simulink model "board_fullstate_lab5"  (R2015a)
settings: Solver=ode3  StartTime=0.0  StopTime=inf  FixedStep=0.001  RelTol=1e-3
undefined symbols (not defined in the file or in its folder): A, frequency, Kx, Kxi, Ky, Kyi, ref, ref_2, ref_3, T1gain, T1offset, T2gain, T2offset, Xtare_raw, Xtare_real, Ytare_raw, Ytare_real
libraries: PoliArd x12, simulink_extras x1, dspsigops x1
settings Model: ExtModeTrigDuration=2  Creator=User  LastModifiedBy=eduar
settings OptimizationCC: OptimizeModelRefInitCode=on  LifeSpan=1
settings DebuggingCC: UnderspecifiedInitializationDetection=Classic  MergeDetectMultiDrivingBlocksExec=none
settings HardwareCC: ProdLargestAtomicInteger=Long  ProdLargestAtomicFloat=Double  ProdEndianess=LittleEndian  ProdHWDeviceType=ARM Compatible->ARM Cortex
settings RTWCC: SystemTargetFile=realtime.tlc  GenerateMakefile=off  TemplateMakefile=realtime.tmf  Description=Run on Target Hardware  RTWVerbose=off
settings ERTTargetCC: CombineOutputUpdateFcns=off  ExtModeTransport=3  ExtModeMexFile=ext_serial_win32_comm_rtt  ExtModeMexArgs=0 1 9600  InlinedParameterPlacement=Hierarchical  ERTSrcFileBannerTemplate=realtime_code_template.cgt  ERTHdrFileBannerTemplate=realtime_code_template.cgt  ERTDataSrcFileTemplate=realtime_code_template.cgt  ERTDataHdrFileTemplate=realtime_code_template.cgt  ERTCustomFileTemplate=realtime_file_process.tlc

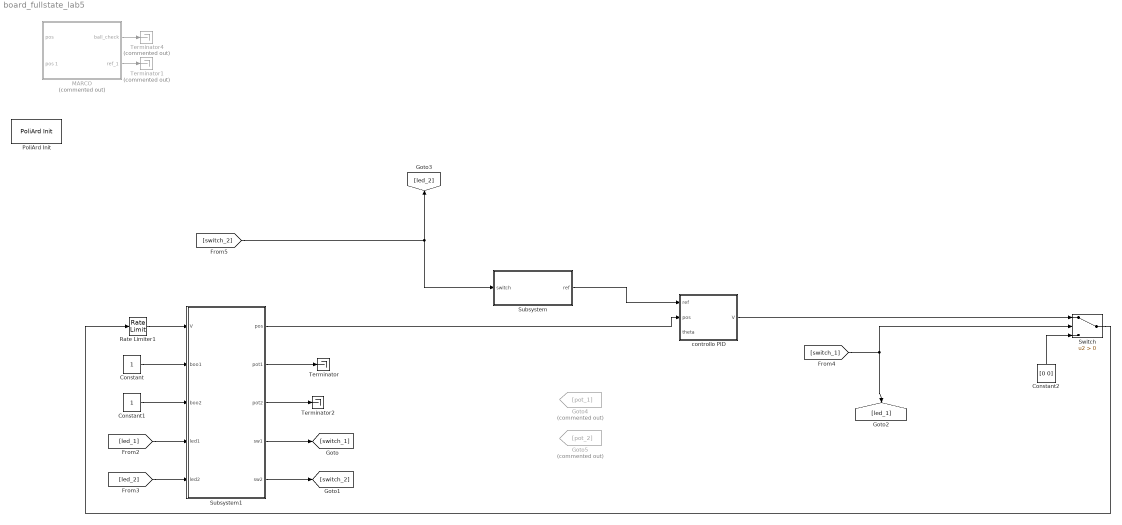
== system board_fullstate_lab5 ==
  Constant : Constant  OutDataTypeStr=boolean  SampleTime=0.01
  Constant1 : Constant  OutDataTypeStr=boolean  SampleTime=0.01
  Constant2 : Constant  Value=[0 0]  SampleTime=0.01
  Goto4 : Goto  Commented=on  GotoTag=pot_1
  Goto5 : Goto  Commented=on  GotoTag=pot_2
  MARCO : Subsystem  Commented=on
  PoliArd Init : PoliArd/PoliArd Init
  Rate Limiter1 : RateLimiter  RisingSlewLimit=20  FallingSlewLimit=-20  SampleTimeMode=inherited
  Subsystem : Subsystem
  Subsystem1 : Subsystem
  Switch : Switch  Criteria=u2 > Threshold
  Terminator : Terminator
  Terminator1 : Terminator  Commented=on
  Terminator2 : Terminator
  Terminator4 : Terminator  Commented=on
  controllo PID : Subsystem  SystemSampleTime=0.01
  wires:
  Subsystem1/1("pos ") -> controllo PID/2("pos ")
  Subsystem1/4(sw1) -> [switch_1]
  Subsystem1/5(sw2) -> [switch_2]
  [led_1] -> Subsystem1/4("led1 ")
  Constant/1 -> Subsystem1/2(boo1)
  Constant1/1 -> Subsystem1/3(boo2)
  [led_2] -> Subsystem1/5(led2)
  MARCO/2(ref_1) -> Terminator1/1
  [switch_1] -> Switch/2, [led_1]
  MARCO/1(ball_check) -> Terminator4/1
  Constant2/1 -> Switch/3
  controllo PID/1(V) -> Switch/1
  Switch/1 -> Rate Limiter1/1
  Rate Limiter1/1 -> Subsystem1/1(V)
  Subsystem1/3(pot2) -> Terminator2/1
  Subsystem1/2(pot1) -> Terminator/1
  [switch_2] -> [led_2], Subsystem/1("switch ")
  Subsystem/1("ref ") -> controllo PID/1("ref ")

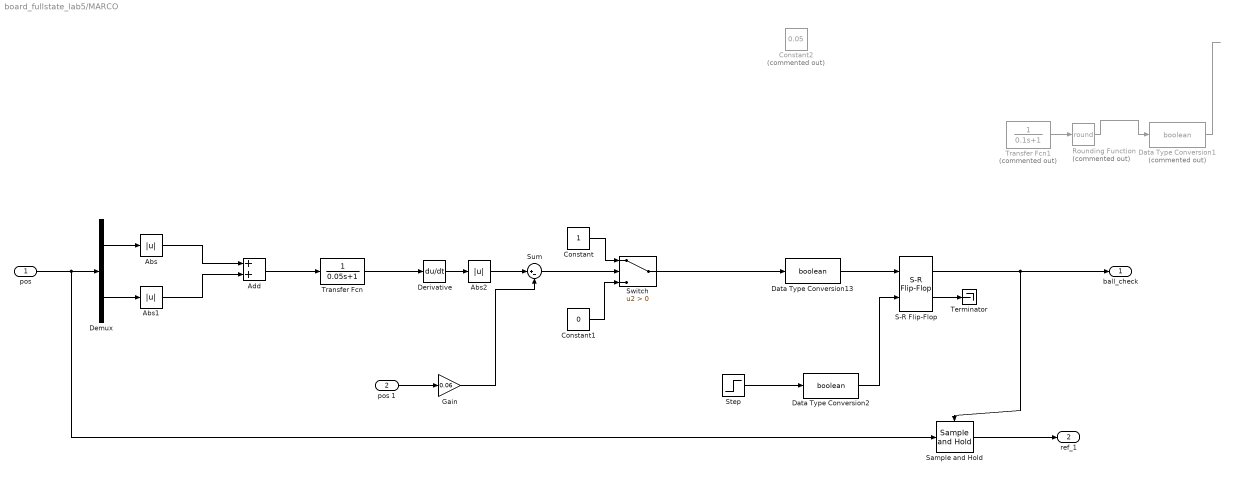
== system board_fullstate_lab5/MARCO ==
  "pos " : Inport
  pos 1 : Inport  Port=2
  Abs : Abs
  Abs1 : Abs
  Abs2 : Abs
  Add : Sum
  Constant : Constant
  Constant1 : Constant  Value=0
  Constant2 : Constant  Commented=on  Value=0.05
  Data Type Conversion1 : DataTypeConversion  Commented=on  OutDataTypeStr=boolean
  Data Type Conversion13 : DataTypeConversion  OutDataTypeStr=boolean
  Data Type Conversion2 : DataTypeConversion  OutDataTypeStr=boolean
  Demux : Demux  Outputs=2
  Derivative : Derivative
  Gain : Gain  Gain=0.06
  Rounding Function : Rounding  Commented=on  Operator=round
  S-R Flip-Flop : simulink_extras/Flip Flops/S-R Flip-Flop  initial_condition=0
  Sample and Hold : dspsigops/Sample and Hold  trig=Rising edge  initCond=0  latchinput=off
  Step : Step  Before=1  After=0
  Sum : Sum  Inputs=|+-
  Switch : Switch  Criteria=u2 > Threshold
  Terminator : Terminator
  Transfer Fcn : TransferFcn  Denominator=[0.05 1]
  Transfer Fcn1 : TransferFcn  Commented=on  Denominator=[0.1 1]
  ball_check : Outport
  ref_1 : Outport  Port=2
  wires:
  "pos "/1 -> Sample and Hold/1, Demux/1
  Demux/1 -> Abs/1
  Demux/2 -> Abs1/1
  Abs1/1 -> Add/2
  Abs/1 -> Add/1
  Derivative/1 -> Abs2/1
  Abs2/1 -> Sum/1
  Sum/1 -> Switch/2
  Constant/1 -> Switch/1
  Constant1/1 -> Switch/3
  Sample and Hold/1 -> ref_1/1
  Add/1 -> Transfer Fcn/1
  Transfer Fcn/1 -> Derivative/1
  Gain/1 -> Sum/2
  S-R Flip-Flop/1 -> ball_check/1, Sample and Hold/Trigger
  S-R Flip-Flop/2 -> Terminator/1
  Data Type Conversion13/1 -> S-R Flip-Flop/1
  Switch/1 -> Data Type Conversion13/1
  Transfer Fcn1/1 -> Rounding Function/1
  Rounding Function/1 -> Data Type Conversion1/1
  ? -> Transfer Fcn1/1
  Data Type Conversion1/1 -> ?
  Data Type Conversion2/1 -> S-R Flip-Flop/2
  Step/1 -> Data Type Conversion2/1
  pos 1/1 -> Gain/1

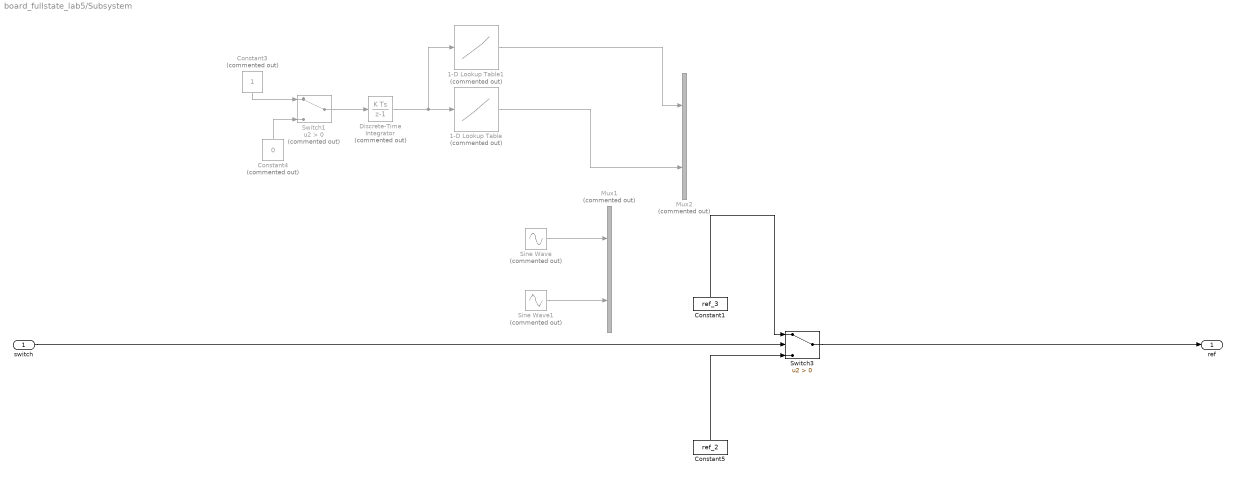
== system board_fullstate_lab5/Subsystem ==
  "switch " : Inport
  1-D Lookup Table : Lookup_n-D  Commented=on  NumberOfTableDimensions=1  BreakpointsForDimension1=ref.y.t  Table=ref.y.v  InternalRulePriority=Speed  RndMeth=Simplest  InputSameDT=on
  1-D Lookup Table1 : Lookup_n-D  Commented=on  NumberOfTableDimensions=1  BreakpointsForDimension1=ref.x.t  Table=ref.x.v  InternalRulePriority=Speed  RndMeth=Simplest  InputSameDT=on
  Constant1 : Constant  Value=ref_3
  Constant3 : Constant  Commented=on
  Constant4 : Constant  Commented=on  Value=0
  Constant5 : Constant  Value=ref_2  SampleTime=0.01
  Discrete-Time Integrator : DiscreteIntegrator  Commented=on  InitialConditionSetting=State (most efficient)  SampleTime=0.01
  Mux1 : Mux  Commented=on  Inputs=2
  Mux2 : Mux  Commented=on  Inputs=2
  Sine Wave : Sin  Commented=on  Amplitude=A  Frequency=frequency  SampleTime=0
  Sine Wave1 : Sin  Commented=on  Amplitude=A  Frequency=frequency  Phase=pi/2  SampleTime=0
  Switch1 : Switch  Commented=on  Criteria=u2 > Threshold
  Switch3 : Switch  Criteria=u2 > Threshold
  "ref " : Outport
  wires:
  Switch1/1 -> Discrete-Time Integrator/1
  Constant3/1 -> Switch1/1
  Constant4/1 -> Switch1/3
  Constant5/1 -> Switch3/3
  Switch3/1 -> "ref "/1
  "switch "/1 -> Switch3/2
  Discrete-Time Integrator/1 -> 1-D Lookup Table1/1, 1-D Lookup Table/1
  Sine Wave/1 -> Mux1/1
  Sine Wave1/1 -> Mux1/2
  1-D Lookup Table1/1 -> Mux2/1
  1-D Lookup Table/1 -> Mux2/2
  Constant1/1 -> Switch3/1

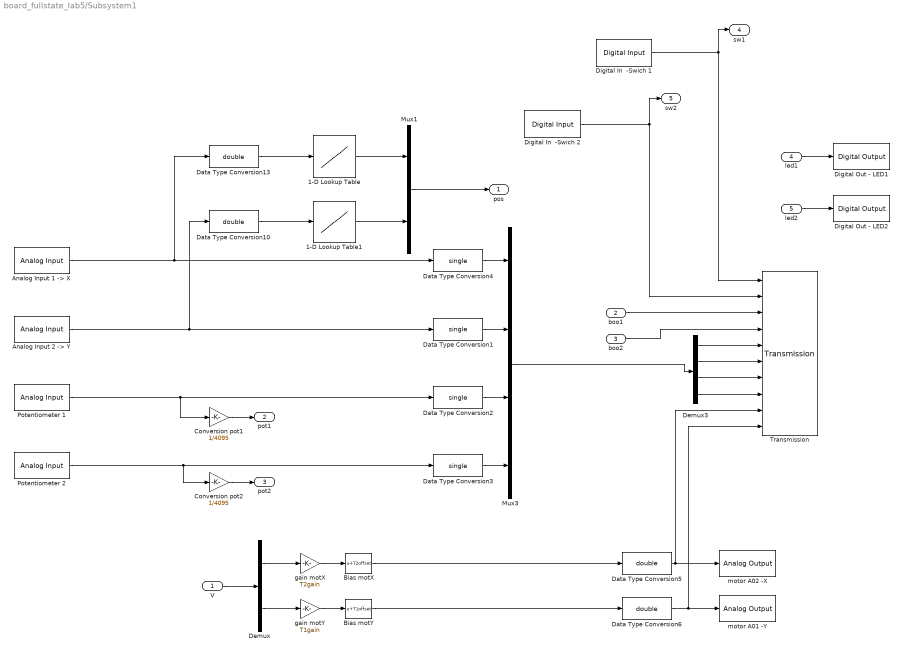
== system board_fullstate_lab5/Subsystem1 ==
  V : Inport
  boo1 : Inport  Port=2
  boo2 : Inport  Port=3
  "led1 " : Inport  Port=4
  led2 : Inport  Port=5
  1-D Lookup Table : Lookup_n-D  NumberOfTableDimensions=1  BreakpointsForDimension1=Xtare_raw  Table=Xtare_real  InternalRulePriority=Speed  RndMeth=Simplest  InputSameDT=on
  1-D Lookup Table1 : Lookup_n-D  NumberOfTableDimensions=1  BreakpointsForDimension1=Ytare_raw  Table=Ytare_real  InternalRulePriority=Speed  RndMeth=Simplest  InputSameDT=on
  "Analog Input 1 -> X" : PoliArd/Analog Input  AIpin_mask=1  AIsample=0.01
  "Analog Input 2 -> Y" : PoliArd/Analog Input  AIpin_mask=2  AIsample=0.01
  Bias motX : Bias  Bias=T2offset
  Bias motY : Bias  Bias=T1offset
  Conversion pot1 : Gain  Gain=1/4095
  Conversion pot2 : Gain  Gain=1/4095
  Data Type Conversion{1..4} (4 alike) : DataTypeConversion  OutDataTypeStr=single
  Data Type Conversion{5..6,10,13} (4 alike) : DataTypeConversion  OutDataTypeStr=double
  Demux : Demux  Outputs=2
  Demux3 : Demux
  Digital In  -Swich 1 : PoliArd/Digital Input  DI_pin=2  DIsample=0.01
  Digital In  -Swich 2 : PoliArd/Digital Input  DI_pin=3  DIsample=0.01
  Digital Out - LED1 : PoliArd/Digital Output  DO_pin=1
  Digital Out - LED2 : PoliArd/Digital Output  DO_pin=2
  Mux1 : Mux  Inputs=2
  Mux3 : Mux
  Potentiometer 1 : PoliArd/Analog Input  AIpin_mask=8  AIsample=-1
  Potentiometer 2 : PoliArd/Analog Input  AIpin_mask=9  AIsample=-1
  Transmission : PoliArd/Transmission  sample_freq=100  sig_to_send=6
  gain motX : Gain  Gain=T2gain
  gain motY : Gain  Gain=T1gain
  motor A01 -Y : PoliArd/Analog Output  DAC_pin_mask=2
  motor A02 -X : PoliArd/Analog Output  DAC_pin_mask=1
  "pos " : Outport
  pot1 : Outport  Port=2
  pot2 : Outport  Port=3
  sw1 : Outport  Port=4
  sw2 : Outport  Port=5
  wires:
  Demux3/3 -> Transmission/7
  Demux3/1 -> Transmission/5
  Demux3/2 -> Transmission/6
  Conversion pot2/1 -> pot2/1
  Potentiometer 2/1 -> Data Type Conversion3/1, Conversion pot2/1
  Conversion pot1/1 -> pot1/1
  Potentiometer 1/1 -> Conversion pot1/1, Data Type Conversion2/1
  boo1/1 -> Transmission/3
  boo2/1 -> Transmission/4
  "led1 "/1 -> Digital Out - LED1/1
  led2/1 -> Digital Out - LED2/1
  Mux1/1 -> "pos "/1
  Digital In  -Swich 1/1 -> Transmission/1, sw1/1
  Digital In  -Swich 2/1 -> sw2/1, Transmission/2
  "Analog Input 1 -> X"/1 -> Data Type Conversion13/1, Data Type Conversion4/1
  "Analog Input 2 -> Y"/1 -> Data Type Conversion10/1, Data Type Conversion1/1
  gain motX/1 -> Bias motX/1
  gain motY/1 -> Bias motY/1
  Demux/1 -> gain motX/1
  Demux/2 -> gain motY/1
  V/1 -> Demux/1
  Demux3/4 -> Transmission/8
  Bias motY/1 -> Data Type Conversion6/1
  Data Type Conversion5/1 -> motor A02 -X/1, Transmission/9
  Data Type Conversion6/1 -> Transmission/10, motor A01 -Y/1
  Bias motX/1 -> Data Type Conversion5/1
  Data Type Conversion13/1 -> 1-D Lookup Table/1
  1-D Lookup Table/1 -> Mux1/1
  Data Type Conversion10/1 -> 1-D Lookup Table1/1
  1-D Lookup Table1/1 -> Mux1/2
  Mux3/1 -> Demux3/1
  Data Type Conversion4/1 -> Mux3/1
  Data Type Conversion1/1 -> Mux3/2
  Data Type Conversion2/1 -> Mux3/3
  Data Type Conversion3/1 -> Mux3/4

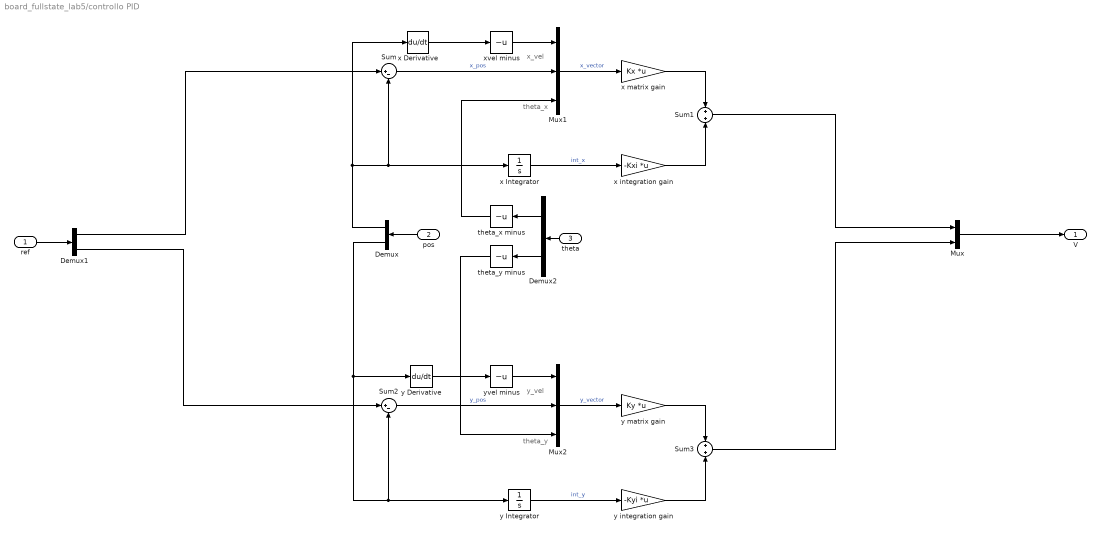
== system board_fullstate_lab5/controllo PID ==
  note: theta_x
  note: x_vel
  note: theta_y
  note: y_vel
  "ref " : Inport
  "pos " : Inport  Port=2
  theta : Inport  Port=3
  Demux : Demux  Outputs=2
  Demux1 : Demux  Outputs=2
  Demux2 : Demux  Outputs=2
  Mux : Mux  Inputs=2
  Mux1 : Mux  Inputs=3
  Mux2 : Mux  Inputs=3
  Sum : Sum  Inputs=|+-
  Sum1 : Sum  Inputs=+|+
  Sum2 : Sum  Inputs=|+-
  Sum3 : Sum  Inputs=+|+
  theta_x minus : UnaryMinus
  theta_y minus : UnaryMinus
  x Derivative : Derivative
  x Integrator : Integrator
  x integration gain : Gain  Gain=-Kxi  Multiplication=Matrix(K*u)
  x matrix gain : Gain  Gain=Kx  Multiplication=Matrix(K*u)
  xvel minus : UnaryMinus
  y Derivative : Derivative
  y Integrator : Integrator
  y integration gain : Gain  Gain=-Kyi  Multiplication=Matrix(K*u)
  y matrix gain : Gain  Gain=Ky  Multiplication=Matrix(K*u)
  yvel minus : UnaryMinus
  V : Outport
  wires:
  "ref "/1 -> Demux1/1
  "pos "/1 -> Demux/1
  Mux/1 -> V/1
  Demux1/1 -> Sum/1
  Demux/1 -> x Integrator/1, Sum/2, x Derivative/1
  x Derivative/1 -> xvel minus/1
  Sum/1 -> Mux1/2  "x_pos"
  Mux1/1 -> x matrix gain/1  "x_vector"
  x Integrator/1 -> x integration gain/1  "int_x"
  x matrix gain/1 -> Sum1/1
  x integration gain/1 -> Sum1/2
  Sum1/1 -> Mux/1
  theta/1 -> Demux2/1
  Demux2/1 -> theta_x minus/1
  y Derivative/1 -> yvel minus/1
  Sum2/1 -> Mux2/2  "y_pos"
  Mux2/1 -> y matrix gain/1  "y_vector"
  y Integrator/1 -> y integration gain/1  "int_y"
  y matrix gain/1 -> Sum3/1
  y integration gain/1 -> Sum3/2
  Demux1/2 -> Sum2/1
  Demux/2 -> y Derivative/1, y Integrator/1, Sum2/2
  Demux2/2 -> theta_y minus/1
  Sum3/1 -> Mux/2
  theta_x minus/1 -> Mux1/3
  theta_y minus/1 -> Mux2/3
  xvel minus/1 -> Mux1/1
  yvel minus/1 -> Mux2/1
